simulink model "SimulinkModelOfCSandItsResponse"  (Simulink 9.1)
settings: Solver=VariableStepAuto  StartTime=0.0  StopTime=10.0  RelTol=1e-3
settings Model: Creator=Dell  LastModifiedBy=Dell
settings DataIOCC: SaveFormat=Dataset
settings OptimizationCC: LifeSpan=auto
settings DebuggingCC: UnderspecifiedInitializationDetection=Simplified  MergeDetectMultiDrivingBlocksExec=error  SFUnexpectedBacktrackingDiag=error  SFNoUnconditionalDefaultTransitionDiag=error  SFExecutionAtInitializationDiag=warning
settings HardwareCC: ProdBitPerPointer=64  ProdBitPerSizeT=64  ProdBitPerPtrDiffT=64  ProdLargestAtomicFloat=Float  ProdIntDivRoundTo=Zero  ProdEndianess=LittleEndian  ProdWordSize=64  ProdHWDeviceType=Intel->x86-64 (Windows64)
settings ModelReferenceCC: PropagateSignalLabelsOutOfModel=on
settings CodeAppCC: StateflowObjectComments=off
settings GRTTargetCC: TargetLangStandard=C99 (ISO)  CombineOutputUpdateFcns=on  GRTInterface=off
settings ConfigComp: CovMetricSettings=dwe  CovHtmlReporting=off  CovSaveCumulativeToWorkspaceVar=off  CovSaveSingleToWorkspaceVar=off  CovExternalEMLEnable=on

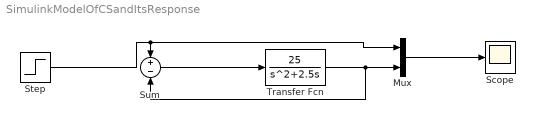
== system SimulinkModelOfCSandItsResponse ==
  Mux : Mux  Inputs=2
  Scope : Scope
  Step : Step  Time=0  SampleTime=0.01
  Sum : Sum  Inputs=+-
  Transfer Fcn : TransferFcn  Numerator=25  Denominator=[1 2.5 0]
  wires:
  Step/1 -> Mux/1, Sum/1
  Sum/1 -> Transfer Fcn/1
  Transfer Fcn/1 -> Sum/2, Mux/2
  Mux/1 -> Scope/1
